simulink model "ML_UAV_3D_2"  (R2018a)
settings: Solver=ode4  StartTime=0.0  StopTime=130  FixedStep=Ts  MaxStep=2*T  MinStep=T  RelTol=1e-4
values from neighbouring files (symbols this model uses):
  Ac = 0.0331    [init_ML_UAV_3D_2.m]
  Am1_LPF = sysd.denominator{1}    [init_ML_UAV_3D_2.m]
  Am2_LPF = sysd.denominator{1}    [init_ML_UAV_3D_2.m]
  Am_coup_LPF = sysd.denominator{1}    [init_ML_UAV_3D_2.m]
  Amp_sf = 3    [init_ML_UAV_3D_2.m]
  Amp_sf_rp = 0.05*uav.m*g    [init_ML_UAV_3D_2.m]
  Bm1_LPF = sysd.numerator{1}    [init_ML_UAV_3D_2.m]
  Bm2_LPF = sysd.numerator{1}    [init_ML_UAV_3D_2.m]
  Bm_coup_LPF = sysd.numerator{1}    [init_ML_UAV_3D_2.m]
  C_S = [5;5;9]*10^-3    [init_ML_UAV_3D_2.m]
  Cd_u = 0.2    [init_ML_UAV_3D_2.m]
  dc_M_p = 6.7    [init_ML_UAV_3D_2.m]
  eps_V = 0.5    [init_ML_UAV_3D_2.m]
  g = 9.81    [init_ML_UAV_3D_2.m]
  gamma_d_p = (2*0.3/0.03*2*0.2*12/4)/10    (= 2.4)    [init_ML_UAV_3D_2.m]
  k3 = 24    [init_ML_UAV_3D_2.m]
  k4 = 0.8    [init_ML_UAV_3D_2.m]
  min_sf = 5    [init_ML_UAV_3D_2.m]
  min_sf_rp = 0.35*uav.m*g    [init_ML_UAV_3D_2.m]
  OMEGA_FILTER_OUTER = 40    [estimation.m]
  T_init = 10    [init_ML_UAV_3D_2.m]
  Tc = 1/500    (= 0.002)    [estimation.m]
  Tg = 1/ 20    (= 0.05)    [estimation.m]
  Tn = 1/500    (= 0.002)    [estimation.m]
  Ts = 1/500    (= 0.002)    [estimation.m]    (also in init_ML_UAV_3D_2.m)
  Tsc = 1/100    (= 0.01)    [estimation.m]
  Tz = 1/500    (= 0.002)    [estimation.m]
  X_GPS_offset = [0.01 0.005]    [estimation.m]
undefined symbols (not defined in the file or in its folder): Am_HPF, Am_LPF, Am_LPF2, an1, an1_v, an2, an3, Bm_HPF, Bm_LPF, Bm_LPF2, bn1, bn1_v, bn2, bn3, buoy, cable, controller, current, D_b, DiscIntNeverNeededParam, F, filters, J_u, K, kd_t, kp_t, L, Light, magnitude, MIL, Phi0, Psi0, R_b, T, Theta0, theta_q_ini, tolerences, torque_corr, uav, Vol_b, water, wave, X0_u
libraries: simulink x48, simulink_extras x10, UAV_Control x4, dspmtrx3 x2, aerolibwind2 x2
(part 1 of 6)
settings Model: Creator=Ahmad  LastModifiedBy=Ahmad
settings SolverCC: InitialStep=T  AlgebraicLoopSolver=LineSearch

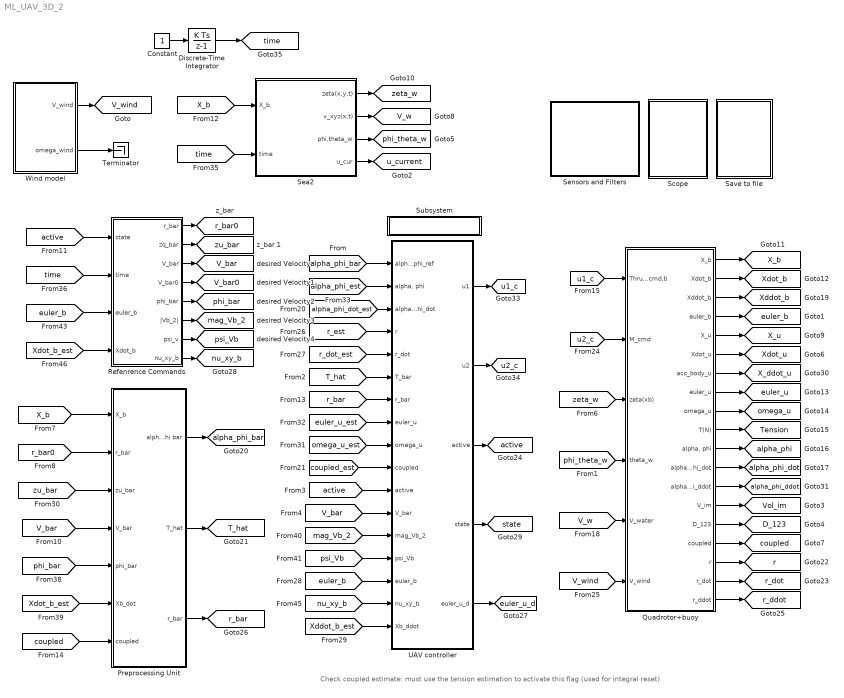
== system ML_UAV_3D_2 ==
  note: Check coupled estimate: must use the tension estimation to activate this flag (used for integral reset)
  Constant : Constant
  Discrete-Time Integrator : DiscreteIntegrator  SampleTime=Ts  ICPrevOutput=DiscIntNeverNeededParam  ICPrevScaledInput=DiscIntNeverNeededParam
  Preprocessing Unit : Subsystem
  Quadrotor+buoy : Subsystem
  Refenrence Commands : Subsystem
  Save to file : Subsystem
  Scope : Subsystem
  Sea2 : Subsystem
  Sensors and Filters : Subsystem
  Subsystem : Subsystem
      settings: OpenFcn=init_ML_UAV_3D_1
      mask Display:
      | text(.5,.5,'load parameters',...
      | 	'horizontalalignment','center');
  Terminator : Terminator
  UAV controller : Subsystem
  Wind model : Subsystem
  tag scope: D_123=global, T_hat=global, Tension=global, V_bar0=global, V_bar=global, V_w=global, V_wind=global, Vol_im=global, X_b=global, X_ddot_u=global, X_u=global, Xddot_b=global, Xdot_b=global, Xdot_u=global, active=global, alpha_phi=global, alpha_phi_bar=global, alpha_phi_ddot=global, alpha_phi_dot=global, coupled=global, euler_b=global, euler_u=global, euler_u_d=global, mag_Vb_2=global, nu_xy_b=global, omega_u=global, phi_bar=global, phi_theta_w=global, psi_Vb=global, r=global, r_bar0=global, r_bar=global, r_ddot=global, r_dot=global, state=global, time=global, u1_c=global, u2_c=global, u_current=global, zeta_w=global, zu_bar=global
  wires:
  [time] -> Sea2/2(time)
  [X_b] -> Sea2/1(X_b)
  Sea2/1(zeta(x,y,t)) -> [zeta_w]
  Sea2/2(v_xyz(x,t)) -> [V_w]
  Sea2/3(phi,theta_w) -> [phi_theta_w]
  [phi_theta_w] -> Quadrotor+buoy/4(theta_w)
  [V_w] -> Quadrotor+buoy/5(V_water)
  [zeta_w] -> Quadrotor+buoy/3(zeta(xb))
  Quadrotor+buoy/5(X_u) -> [X_u]
  Quadrotor+buoy/1(X_b) -> [X_b]
  Quadrotor+buoy/2(Xdot_b) -> [Xdot_b]
  Quadrotor+buoy/8(euler_u) -> [euler_u]
  Quadrotor+buoy/9(omega_u) -> [omega_u]
  Quadrotor+buoy/10(T(N)) -> [Tension]
  Quadrotor+buoy/11("alpha, phi") -> [alpha_phi]
  Quadrotor+buoy/12("alpha_dot, phi_dot") -> [alpha_phi_dot]
  [X_b] -> Preprocessing Unit/1(X_b)
  Preprocessing Unit/1("alpha, phi bar") -> [alpha_phi_bar]
  Preprocessing Unit/2(T_hat) -> [T_hat]
  Quadrotor+buoy/3(Xddot_b) -> [Xddot_b]
  Quadrotor+buoy/4(euler_b) -> [euler_b]
  Quadrotor+buoy/6(Xdot_u) -> [Xdot_u]
  Sea2/4(u_cur) -> [u_current]
  Quadrotor+buoy/14(V_im) -> [Vol_im]
  Quadrotor+buoy/15(D_123) -> [D_123]
  [alpha_phi_bar] -> UAV controller/1(alpha_phi_ref)
  [alpha_phi_est] -> UAV controller/2("alpha, phi")
  [alpha_phi_dot_est] -> UAV controller/3(alpha_phi_dot)
  [T_hat] -> UAV controller/6(T_bar)
  [Xddot_b_est] -> UAV controller/17(Xb_ddot)
  [euler_u_est] -> UAV controller/8(euler_u)
  [omega_u_est] -> UAV controller/9(omega_u)
  Quadrotor+buoy/16(coupled) -> [coupled]
  [active] -> Refenrence Commands/1(state)
  [r_bar] -> UAV controller/7(r_bar)
  Quadrotor+buoy/17(r) -> [r]
  Quadrotor+buoy/18(r_dot) -> [r_dot]
  [r_est] -> UAV controller/4(r)
  UAV controller/3(" active") -> [active]
  [active] -> UAV controller/11(active)
  [coupled_est] -> UAV controller/10(coupled)
  Quadrotor+buoy/19(r_ddot) -> [r_ddot]
  [r_dot_est] -> UAV controller/5(r_dot)
  Preprocessing Unit/3(" r_bar") -> [r_bar]
  UAV controller/4(state) -> [state]
  Quadrotor+buoy/7(acc_body_u) -> [X_ddot_u]
  Quadrotor+buoy/13("alpha_ddot, phi_ddot") -> [alpha_phi_ddot]
  Wind model/1(V_wind) -> [V_wind]
  Wind model/2(omega_wind) -> Terminator/1
  [V_wind] -> Quadrotor+buoy/6(V_wind)
  Refenrence Commands/1(r_bar) -> [r_bar0]
  [r_bar0] -> Preprocessing Unit/2(r_bar)
  Refenrence Commands/4(V_bar0) -> [V_bar0]
  Refenrence Commands/3(V_bar) -> [V_bar]
  [V_bar] -> Preprocessing Unit/4(V_bar)
  UAV controller/1(u1) -> [u1_c]
  UAV controller/2(u2) -> [u2_c]
  [u1_c] -> Quadrotor+buoy/1(Thrust_cmd,b)
  [u2_c] -> Quadrotor+buoy/2(M_cmd)
  Refenrence Commands/2(zq_bar) -> [zu_bar]
  [zu_bar] -> Preprocessing Unit/3(zu_bar)
  Constant/1 -> Discrete-Time Integrator/1
  Discrete-Time Integrator/1 -> [time]
  [time] -> Refenrence Commands/2(time)
  Refenrence Commands/5("phi_bar ") -> [phi_bar]
  [phi_bar] -> Preprocessing Unit/5(phi_bar)
  [Xdot_b_est] -> Preprocessing Unit/6(Xb_dot)
  Refenrence Commands/7(psi_v) -> [psi_Vb]
  Refenrence Commands/6(|Vb_2|) -> [mag_Vb_2]
  UAV controller/5(euler_u_d) -> [euler_u_d]
  [coupled] -> Preprocessing Unit/7(coupled)
  [psi_Vb] -> UAV controller/14(psi_Vb)
  [mag_Vb_2] -> UAV controller/13(mag_Vb_2)
  [euler_b] -> UAV controller/15(euler_b)
  [euler_b] -> Refenrence Commands/3(euler_b)
  Refenrence Commands/8(nu_xy_b) -> [nu_xy_b]
  [Xdot_b_est] -> Refenrence Commands/4(Xdot_b)
  [nu_xy_b] -> UAV controller/16(nu_xy_b)
  [V_bar] -> UAV controller/12(V_bar)

== system ML_UAV_3D_2/Preprocessing Unit ==
  X_b : Inport
  r_bar : Inport  Port=2
  zu_bar : Inport  Port=3
  V_bar : Inport  Port=4
  phi_bar : Inport  Port=5
  Xb_dot : Inport  Port=6
  coupled : Inport  Port=7
  Constant : Constant  Value=0
  Constant1 : Constant  Value=buoy.b_11
  Constant2 : Constant  Value=water.rho
  Constant3 : Constant  Value=water.nu
  Damping Coefficient Calculation : MATLAB Function  TreatAsAtomicUnit=on
  Dh @ no tension : Constant  Value=buoy.Delta_h
  Discrete Transfer Fcn1 : DiscreteTransferFcn  Numerator=filters.BmZ_LPF  Denominator=filters.AmZ_LPF  InitialStates=[1 1]*(1-sum(filters.AmZ_LPF))/(sum(filters.BmZ_LPF))*buoy.X0(3)
  Display : Display
  Display1 : Display
  Mux : Mux  Inputs=3
  Mux1 : Mux  Inputs=2
  Saturation : Saturate  UpperLimit=inf  LowerLimit=tolerences.epsilon_1
  Sum : Sum  Inputs=|+-
  Switch : Switch  Criteria=u2 > Threshold
  V_bar2 : InportShadow  Port=4
  alpha act vs des {,1..3} (4 alike) : Scope
  bottom plan : Constant  Value=buoy.h
  bottom plan1 : Constant  Value=buoy.l
  buoy elvation : Scope
  r_bar1 : InportShadow  Port=2
  "setpoint velocity controller " : MATLAB Function  TreatAsAtomicUnit=on
  smooth lower bound1 : Subsystem
  z_b : Selector  InputPortWidth=3  IndexOptions=Index vector (dialog)  Indices=3  OutputSizes=1
  "alpha, phi bar" : Outport
  T_hat : Outport  Port=2
  " r_bar" : Outport  Port=3
  wires:
  X_b/1 -> z_b/1
  zu_bar/1 -> alpha act vs des 1/1, "setpoint velocity controller "/6(zu_ref)
  Mux/1 -> buoy elvation/1
  Sum/1 -> Mux/3
  z_b/1 -> Discrete Transfer Fcn1/1, Mux/1, Sum/1
  Discrete Transfer Fcn1/1 -> "setpoint velocity controller "/5(zb), Mux/2, Sum/2  "better"
  r_bar1/1 -> " r_bar"/1
  Mux1/1 -> "alpha act vs des "/1, "alpha, phi bar"/1
  "setpoint velocity controller "/2(phi_bar_dec) -> Mux1/2
  [D11_0] -> "setpoint velocity controller "/7(D_b11)
  "setpoint velocity controller "/1(alpha_ref) -> Mux1/1
  phi_bar/1 -> alpha act vs des 3/1, "setpoint velocity controller "/2(phi_bar)
  V_bar/1 -> "setpoint velocity controller "/1(V_ref)
  Xb_dot/1 -> "setpoint velocity controller "/3(Vb)
  Saturation/1 -> smooth lower bound1/1(u)
  "setpoint velocity controller "/3(T_bar) -> Saturation/1
  smooth lower bound1/1(sat(u)) -> Switch/1
  Damping Coefficient Calculation/3(D11_0) -> [D11_0]
  Constant2/1 -> Damping Coefficient Calculation/5(rho)
  Constant1/1 -> Damping Coefficient Calculation/7(b_11)
  bottom plan/1 -> Damping Coefficient Calculation/3(h_b)
  bottom plan1/1 -> Damping Coefficient Calculation/4(l_b)
  Dh @ no tension/1 -> Damping Coefficient Calculation/2(delta_h)
  V_bar2/1 -> Damping Coefficient Calculation/1(V_bar)
  Constant3/1 -> Damping Coefficient Calculation/6(nu)
  r_bar/1 -> alpha act vs des 2/1, "setpoint velocity controller "/4(r_ref)
  Damping Coefficient Calculation/1(Re) -> Display/1
  Damping Coefficient Calculation/2(C_S_bar) -> Display1/1
  coupled/1 -> Switch/2
  Switch/1 -> T_hat/1
  Constant/1 -> Switch/3

== system ML_UAV_3D_2/Quadrotor+buoy ==
  Thrust_cmd,b : Inport
  M_cmd : Inport  Port=2
  zeta(xb) : Inport  Port=3
  theta_w : Inport  Port=4
  V_water : Inport  Port=5
  V_wind : Inport  Port=6
  6-DOF equations of motion Earth frame : Subsystem  mask(3DOF EoM, earth frame){pos_b_ini=buoy.X0, pos_u_ini=uav.X0, euler_b_ini=0, a_p_0=[uav.alpha_0; uav.phi_0], v_b_ini=buoy.V0, v_u_ini=uav.V0, euler_u_ini=uav.euler_0, omega_u_ini=0, m_u=1.7, J_u=uav.J, h_b=buoy.h, l_b=buoy.l, m_b=buoy.m, J_b=buoy.J, a_ii=[buoy.a_11 buoy.a_22  buoy.a_33], b_ii=[buoy.b_11 buoy.b_22 buoy.b_33 0 0 0], L=cable.L_0, g=g, rho_w=water.rho, coupled_ini=off}
      mask prompts: pos_b_ini "Buoy initial position (x y z):"; pos_u_ini "UAV initial position (x y z):"; euler_b_ini "Buoy initial body attitude:"; a_p_0 "Cable initial angle:"; v_b_ini "Buoy initial velocity (x y z):"; v_u_ini "UAV initial velocity (x y z):"; euler_u_ini "Quadrotor initial body attitude (quadrotor):"; omega_u_ini "Quadrotor initial body rotation rate:"; m_u "Quadrotor mass:"; J_u "Quadrotor moment of Inertia (3x3):"; h_b "Buoy height:"; l_b "Buoy lenght:"; m_b "Buoy mass:"; J_b "Buoy moment of Inertia (3x3):"; a_ii "Added mass (1x6):"; b_ii "Buoy damping coefficients (1x6):"; L "Cable length:"; g "gravity:"; rho_w "water density:"; coupled_ini "Initial coupling state (checked for coupled)"
      mask init:
      | nu_w = 1.787*10^-6;   % kinematic viscosity of water (m2/s)
      | g = 9.81;               % gravity constant (m/s2)
      | rho_w = 1000;   % water density (kg/m3)
      | rho_a = 1.225;             % air density (kg/m^3)
      | 
      | r_0 = norm(pos_u_ini - pos_b_ini);
      | 
      | R_S2C_0 = [cos(a_p_0(1))*cos(a_p_0(2))  -sin(a_p_0(1))*cos(a_p_0(2)) -sin(a_p_0(2))
      |            cos(a_p_0(1))*sin(a_p_0(2))  -sin(a_p_0(1))*sin(a_p_0(2))  cos(a_p_0(2))
      |            sin(a_p_0(1))                 cos(a_p_0(1))                0            ];
      |        
      | pos_u_0_coupled = pos_b_ini+L*[cos(a_p_0(1))*cos(a_p_0(2)); cos(a_p_0(1))*sin(a_p_0(2)); sin(a_p_0(1))];
      mask Display:
      | port_label('input',1,'u_1 (N)','texmode','on');
      | port_label('input',2,'\tau_{u,r} (N.m)','texmode','on');
      | port_label('input',3,'\zeta (m)','texmode','on');
      | port_label('input',4,'\phi_w,\theta_w (rad)','texmode','on');
      | port_label('input',5,'V_{water} (m/s)','texmode','on');
      | port_label('input',6,'V_{wind} (m/s)','texmode','on');
      | 
      | port_label('output',1,'X_b (m)','texmode','on');
      | port_label('output',2,'X_{b,dot} (m/s)','texmode','on');
      | port_label('output',3,'X_{b,ddot} (m/s)','texmode','on');
      | port_label('output',4,'euler_b(rad)','texmode','on');
      | port_label('output',5,'X_u (m)','texmode','on');
      | port_label('output',6,'X_{u,dot} (m/s)','texmode','on');
      | port_label('output',7,'X_{u,ddot} (m/s^2)','texmode','on');
      | port_label('output',8,'euler_u(rad)','texmode','on');
      | port_label('output',9,'\omega_u (rad/s)','texmode','on');
      | port_label('output',10,'\alpha, \phi (rad)','texmode','on');
      | port_label('output',11,'\alpha_{dot} \phi_{dot} (rad/s)','texmode','on');
      | port_label('output',12,'\alpha_{ddot} \phi_{ddot} (rad/s)','texmode','on');
      | port_label('output',13,'r (m)','texmode','on');
      | port_label('output',14,'r_{dot} (m/s)','texmode','on');
      | port_label('output',15,'r_{ddot} (m/s)','texmode','on');
      | port_label('output',16,'T (N)','texmode','on');
      | port_label('output',17,'V_{im} (m^3)','texmode','on');
      | port_label('output',18,'D_{123}','texmode','on');
      | port_label('output',19,'coupled','texmode','on');
  Gain : Gain
  Gain1 : Gain  Gain=[1 1 1]
  Mux : Mux  Inputs=2
  Mux1 : Mux  Inputs=2
  Saturation - Limit Height Controller1 : Saturate  UpperLimit=uav.K*uav.L*uav.torque_corr*[1 1 1]  LowerLimit=-uav.K*uav.L*uav.torque_corr*[1 1 1]
  Saturation - Limit Height Controller3 : Saturate  UpperLimit=uav.n_motors*uav.K  LowerLimit=0
  Signal Specification{,1..6,8} (8 alike) : SignalSpecification  Dimensions=[3,1]
  Signal Specification10 : SignalSpecification  Dimensions=[2,1]
  Signal Specification7 : SignalSpecification  Dimensions=[2,1]
  Signal Specification9 : SignalSpecification  Dimensions=[2,1]
  Torque : Scope
  "Xb " : Scope
  "Xq " : Scope
  motor dynamics (thrust) : DiscreteTransferFcn  Numerator=filters.Bm  Denominator=filters.Am  InitialStates=-filters.Am(2)/filters.Bm(2)*uav.m*g/cos(uav.euler_0(2))
  motor dynamics (torque) : DiscreteTransferFcn  Numerator=filters.Bm  Denominator=filters.Am
  thrust : Scope
  X_b : Outport
  Xdot_b : Outport  Port=2
  Xddot_b : Outport  Port=3
  euler_b : Outport  Port=4
  X_u : Outport  Port=5
  Xdot_u : Outport  Port=6
  acc_body_u : Outport  Port=7
  euler_u : Outport  Port=8
  omega_u : Outport  Port=9
  T(N) : Outport  Port=10
  "alpha, phi" : Outport  Port=11
  "alpha_dot, phi_dot" : Outport  Port=12
  "alpha_ddot, phi_ddot" : Outport  Port=13
  V_im : Outport  Port=14
  D_123 : Outport  Port=15
  coupled : Outport  Port=16
  r : Outport  Port=17
  r_dot : Outport  Port=18
  r_ddot : Outport  Port=19
  tag scope: tau_ur=global, u1=global
  wires:
  Saturation - Limit Height Controller3/1 -> Gain/1, Mux/2
  motor dynamics (torque)/1 -> Saturation - Limit Height Controller1/1
  M_cmd/1 -> Mux1/1, motor dynamics (torque)/1
  Thrust_cmd,b/1 -> Mux/1, motor dynamics (thrust)/1
  Saturation - Limit Height Controller1/1 -> Mux1/2, Gain1/1
  zeta(xb)/1 -> 6-DOF equations of motion Earth frame/3(zeta)
  theta_w/1 -> 6-DOF equations of motion Earth frame/4(phi_theta_w)
  V_water/1 -> 6-DOF equations of motion Earth frame/5(V_w)
  6-DOF equations of motion Earth frame/5(Xu) -> Signal Specification3/1  "X_u"
  6-DOF equations of motion Earth frame/1(Xb) -> Signal Specification/1  "X_b"
  6-DOF equations of motion Earth frame/2(Xb_dot) -> Signal Specification1/1  "Xdot_b"
  6-DOF equations of motion Earth frame/6(Xu_dot) -> Signal Specification4/1  "V_u"
  6-DOF equations of motion Earth frame/4(Attitude_buoy) -> euler_b/1  "euler_b"
  6-DOF equations of motion Earth frame/8(Attitude_quadrotor) -> Signal Specification6/1  "euler_u"
  6-DOF equations of motion Earth frame/9(omega_quadrotor) -> Signal Specification8/1  "omega_u"
  6-DOF equations of motion Earth frame/3(Xb_ddot) -> Signal Specification2/1
  motor dynamics (thrust)/1 -> Saturation - Limit Height Controller3/1
  6-DOF equations of motion Earth frame/11(alpha_phi_dot) -> Signal Specification9/1  "alpha_dot"
  6-DOF equations of motion Earth frame/16(Cable Tension) -> T(N)/1  "tension"
  6-DOF equations of motion Earth frame/10(alpha_phi) -> Signal Specification7/1  "alpha"
  Mux/1 -> thrust/1
  Mux1/1 -> Torque/1
  6-DOF equations of motion Earth frame/17(V_im) -> V_im/1
  Gain/1 -> 6-DOF equations of motion Earth frame/1(u1), [u1]
  Gain1/1 -> 6-DOF equations of motion Earth frame/2(tau_ur), [tau_ur]
  6-DOF equations of motion Earth frame/18("D_123 ") -> D_123/1
  6-DOF equations of motion Earth frame/19(coupled) -> coupled/1
  6-DOF equations of motion Earth frame/13("  r") -> r/1
  6-DOF equations of motion Earth frame/14("  rdot") -> r_dot/1
  6-DOF equations of motion Earth frame/15("  rddot") -> r_ddot/1
  6-DOF equations of motion Earth frame/7(Xu_ddot) -> Signal Specification5/1
  6-DOF equations of motion Earth frame/12(alpha_ddot) -> Signal Specification10/1
  V_wind/1 -> 6-DOF equations of motion Earth frame/6(V_wind)
  Signal Specification/1 -> "Xb "/1, X_b/1
  Signal Specification2/1 -> Xddot_b/1
  Signal Specification1/1 -> Xdot_b/1
  Signal Specification3/1 -> "Xq "/1, X_u/1
  Signal Specification5/1 -> acc_body_u/1
  Signal Specification4/1 -> Xdot_u/1
  Signal Specification6/1 -> euler_u/1
  Signal Specification8/1 -> omega_u/1
  Signal Specification7/1 -> "alpha, phi"/1
  Signal Specification10/1 -> "alpha_ddot, phi_ddot"/1
  Signal Specification9/1 -> "alpha_dot, phi_dot"/1

== system ML_UAV_3D_2/Refenrence Commands ==
  note: maybe you should start controlling the velocity imediatly and not wait for the uav to position itself in the expected final azimuth angleeventually the final azimuth angle could change and it is not efficient to follow it from the beginning.let the outer loop velocity controller work by itself.
  note: Smooth reference signals
  note: Initialization phase, reference r and zu
  note: Saturation protection
  note: V_r0_bar is the velocity of the buoy relative
      | to the water current (wave velocity is not included)
  state : Inport
  time : Inport  Port=2
  euler_b : Inport  Port=3
  Xdot_b : Inport  Port=4
  "  Vbar  " : Scope
  "  c" : Scope
  " r_ref " : Constant  Value=[uav.r_0 uav.r_bar]
  Bias : Bias  Bias=water.H+buoy.h/2
  Bias1 : Bias  Bias=-water.H-buoy.h/2
  Constant : Constant  Value=water.H
  Discrete Transfer Fcn (with initial outputs)1 : simulink_extras/Additional Discrete/Discrete Transfer Fcn (with initial outputs)  N=filters.Bm_rref_LPF  D=filters.Am_rref_LPF  U0=0  Y0=uav.r_0  TS=-1
      settings: SourceProductName=Simulink  SourceProductBaseCode=SL
  Discrete Transfer Fcn (with initial outputs)2 : simulink_extras/Additional Discrete/Discrete Transfer Fcn (with initial outputs)  N=filters.BmPsiV_LPF  D=filters.AmPsiV_LPF  U0=uav.phi_0  Y0=uav.phi_0  TS=-1
      settings: SourceProductName=Simulink  SourceProductBaseCode=SL
  Discrete Transfer Fcn (with initial outputs)3 : simulink_extras/Additional Discrete/Discrete Transfer Fcn (with initial outputs)  N=filters.BmV_LPF  D=filters.AmV_LPF  U0=0  Y0=0  TS=-1
      settings: SourceProductName=Simulink  SourceProductBaseCode=SL
  Discrete Transfer Fcn (with initial outputs)4 : simulink_extras/Additional Discrete/Discrete Transfer Fcn (with initial outputs)  N=filters.Bm_rref20_LPF  D=filters.Am_rref20_LPF  U0=0  Y0=uav.r_0  TS=-1
      settings: SourceProductName=Simulink  SourceProductBaseCode=SL
  From File : FromFile  Commented=on  FileName=Export\with waves\SVC\V_bar.mat  SampleTime=0
  From File1 : FromFile  Commented=on  FileName=Export\no waves\SVC\V_bar.mat  SampleTime=0
  From File2 : FromFile  Commented=on  FileName=Export\Monte Carlo\CM_21\SVCS\V_bar.mat  SampleTime=0
  Manual Switch1 : ManualSwitch  CurrentSetting=0
  Manual Switch2 : ManualSwitch  Commented=on
  Manual Switch4 : ManualSwitch
  Mux1 : Mux  Inputs=2
  Mux3 : Mux  Inputs=3
  "Rate Limiter for fly over test " : RateLimiter  RisingSlewLimit=2.5/10  FallingSlewLimit=-2.5/10  SampleTimeMode=inherited
  Saturation Dynamic : simulink/Discontinuities/Saturation Dynamic  OutMin=[]  OutMax=[]  OutDataTypeStr=Inherit: Same as second input  OutDataType=fixdt(1, 16)  OutScaling=2^-10  DoSatur=off
  Saturation Dynamic1 : simulink/Discontinuities/Saturation Dynamic  OutMin=[]  OutMax=[]  OutDataTypeStr=Inherit: Same as second input  OutDataType=fixdt(1, 16)  OutScaling=2^-10  DoSatur=off
  Scope1 : Scope
  Scope2 : Scope
  Selector1 : Selector  InputPortWidth=3  IndexOptions=Index vector (dialog)  Indices=[1,2]  OutputSizes=1
  Switch : Switch  Criteria=u2 > Threshold
  Switch4 : Switch  Criteria=u2 > Threshold
  V_ref : Constant  Value=[5 0+5 -5+10]
  cable length : Constant  Value=cable.L_0
  initialize r_bar : Step  Time=20  SampleTime=0
  minimum velocity error : Constant
  "psi_b " : Selector  InputPortWidth=3  IndexOptions=Index vector (dialog)  Indices=3  OutputSizes=1
  psi_v_ref : Constant  Value=[uav.phi_0*0 pi/2 pi]
  r error threshold [m] : Constant  Value=0.05
  r_ref for the coupled case (pulling) : Constant  Value=cable.L_0
  referense signals selector : MATLAB Function  TreatAsAtomicUnit=on
  setpoint velocity controller1 : MATLAB Function  TreatAsAtomicUnit=on
  smooth z_bar : simulink_extras/Additional Discrete/Discrete Transfer Fcn (with initial outputs)  N=filters.Bm_rref_LPF  D=filters.Am_rref_LPF  U0=uav.X0(3)-0.015  Y0=uav.X0(3)-0.015  TS=-1
      settings: SourceProductName=Simulink  SourceProductBaseCode=SL
  tr ref : Constant  Value=[0 1]
  tv_ref : Constant  Value=[T_init T_init+25 T_init+25+20]
  vector magnitude and angle1 : MATLAB Function  TreatAsAtomicUnit=on
  zu_ref : Constant  Value=[uav.X0(3)-0.015 uav.z_bar]
  r_bar : Outport
  zq_bar : Outport  Port=2
  V_bar : Outport  Port=3
  V_bar0 : Outport  Port=4
  "phi_bar " : Outport  Port=5
  |Vb_2| : Outport  Port=6
  psi_v : Outport  Port=7
  nu_xy_b : Outport  Port=8
  wires:
  referense signals selector/1(V_ref_out) -> setpoint velocity controller1/5(V0_bar), Mux3/3, V_bar0/1
  r_ref for the coupled case (pulling)/1 -> Switch/1, Saturation Dynamic1/1
  referense signals selector/3(r_ref_out) -> Switch/3  "r_ref when not 'pulling'"
  state/1 -> Switch/2
  Saturation Dynamic/1 -> Bias1/1, zq_bar/1
  Constant/1 -> Saturation Dynamic/3
  Bias/1 -> Saturation Dynamic/1
  Saturation Dynamic1/1 -> r_bar/1
  Bias1/1 -> Saturation Dynamic1/3
  smooth z_bar/1 -> Saturation Dynamic/2
  Switch4/1 -> Bias/1, Saturation Dynamic1/2  "r_bar"
  referense signals selector/4(zu_ref_out) -> smooth z_bar/1
  Switch/1 -> Discrete Transfer Fcn (with initial outputs)1/1, Discrete Transfer Fcn (with initial outputs)4/1
  minimum velocity error/1 -> setpoint velocity controller1/1(eps)
  [r_est] -> setpoint velocity controller1/2(r)
  r error threshold [m]/1 -> setpoint velocity controller1/3(er_thr)
  cable length/1 -> setpoint velocity controller1/4(Lc0)
  Xdot_b/1 -> Selector1/1
  setpoint velocity controller1/3(c) -> "  c"/1
  Discrete Transfer Fcn (with initial outputs)3/1 -> Manual Switch1/2, Mux3/1
  Mux3/1 -> "  Vbar  "/1
  initialize r_bar/1 -> Switch4/2
  Discrete Transfer Fcn (with initial outputs)4/1 -> Switch4/1
  Discrete Transfer Fcn (with initial outputs)1/1 -> Switch4/3
  Manual Switch1/1 -> V_bar/1
  From File/1 -> Manual Switch2/2
  From File1/1 -> Manual Switch2/1
  Manual Switch4/1 -> Discrete Transfer Fcn (with initial outputs)3/1, Mux3/2
  setpoint velocity controller1/1(V_bar_out) -> "Rate Limiter for fly over test "/1, Manual Switch4/1
  "Rate Limiter for fly over test "/1 -> Manual Switch4/2
  From File2/1 -> Manual Switch1/1
  time/1 -> referense signals selector/7(t)
  " r_ref "/1 -> referense signals selector/4(r_ref)
  tr ref/1 -> referense signals selector/6(tr_ref)
  zu_ref/1 -> referense signals selector/5(zu_ref)
  tv_ref/1 -> referense signals selector/3(tv_ref)
  V_ref/1 -> referense signals selector/1(V_ref)
  psi_v_ref/1 -> referense signals selector/2(phi_ref)
  referense signals selector/2(phi_ref_out) -> setpoint velocity controller1/6(phi0_bar)
  Selector1/1 -> Scope1/1, vector magnitude and angle1/1(U2)
  vector magnitude and angle1/2(direction2) -> Scope2/1, psi_v/1
  setpoint velocity controller1/2(phi_bar_out) -> Discrete Transfer Fcn (with initial outputs)2/1
  Discrete Transfer Fcn (with initial outputs)2/1 -> "phi_bar "/1
  euler_b/1 -> "psi_b "/1
  "psi_b "/1 -> vector magnitude and angle1/2(psi_b)
  vector magnitude and angle1/3(nu_xb) -> setpoint velocity controller1/7(V), Mux1/1
  vector magnitude and angle1/4(nu_yb) -> Mux1/2
  Mux1/1 -> nu_xy_b/1
  vector magnitude and angle1/1(mag_u2) -> |Vb_2|/1

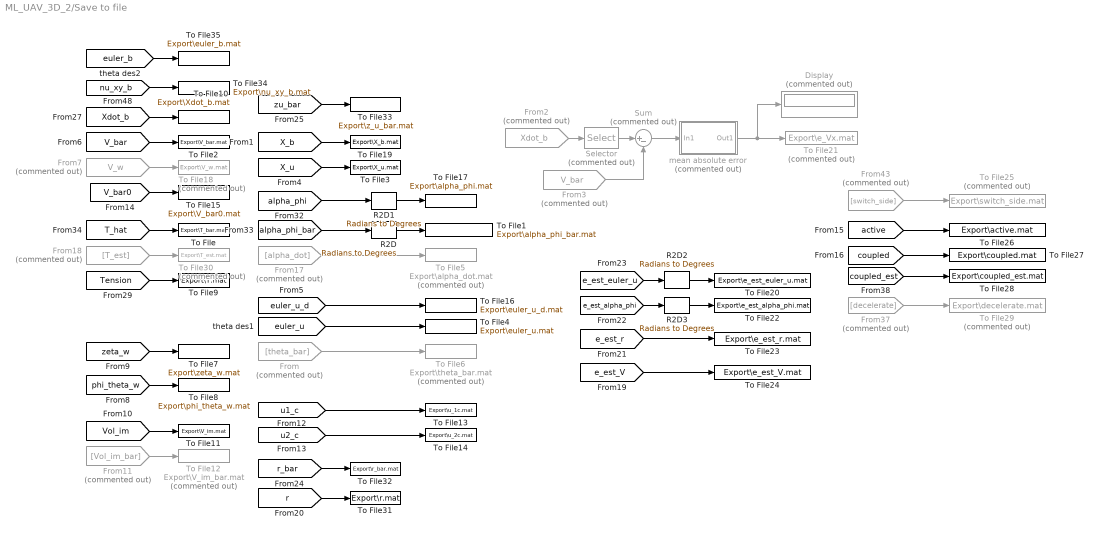
== system ML_UAV_3D_2/Save to file ==
  Display : Display  Commented=on
  From : From  Commented=on  GotoTag=theta_bar  TagVisibility=global
  From11 : From  Commented=on  GotoTag=Vol_im_bar
  From17 : From  Commented=on  GotoTag=alpha_dot  TagVisibility=global
  From18 : From  Commented=on  GotoTag=T_est
  From2 : From  Commented=on  GotoTag=Xdot_b  TagVisibility=global
  From3 : From  Commented=on  GotoTag=V_bar  TagVisibility=global
  From37 : From  Commented=on  GotoTag=decelerate  TagVisibility=global
  From43 : From  Commented=on  GotoTag=switch_side
  From7 : From  Commented=on  GotoTag=V_w  TagVisibility=global
  R2D{,1..3} (4 alike) : simulink_extras/Transformations/Radians to Degrees
  Selector : Selector  Commented=on  InputPortWidth=2  IndexOptions=Index vector (dialog)  Indices=1  OutputSizes=1
  Sum : Sum  Commented=on  Inputs=|+-
  To File : ToFile  Filename=Export\T_bar.mat  MatrixName=T_bar  SaveFormat=Timeseries  SampleTime=floor(Ts/4)
  To File1 : ToFile  Filename=Export\alpha_phi_bar.mat  MatrixName=alpha_phi_bar  SaveFormat=Timeseries  SampleTime=floor(Ts/4)
  To File10 : ToFile  Filename=Export\Xdot_b.mat  MatrixName=Xdot_b  SaveFormat=Timeseries  SampleTime=floor(Ts/4)
  To File11 : ToFile  Filename=Export\V_im.mat  MatrixName=V_im  SaveFormat=Timeseries  SampleTime=floor(Ts/4)
  To File12 : ToFile  Commented=on  Filename=Export\V_im_bar.mat  MatrixName=V_im_bar  SaveFormat=Timeseries  SampleTime=floor(Ts/4)
  To File13 : ToFile  Filename=Export\u_1c.mat  MatrixName=u_1c  SaveFormat=Timeseries  SampleTime=floor(Ts/4)
  To File14 : ToFile  Filename=Export\u_2c.mat  MatrixName=u_2c  SaveFormat=Timeseries  SampleTime=floor(Ts/4)
  To File15 : ToFile  Filename=Export\V_bar0.mat  MatrixName=V_bar0  SaveFormat=Timeseries  SampleTime=floor(Ts/4)
  To File16 : ToFile  Filename=Export\euler_u_d.mat  MatrixName=euler_u_d  SaveFormat=Timeseries  SampleTime=floor(Ts/4)
  To File17 : ToFile  Filename=Export\alpha_phi.mat  MatrixName=alpha_phi  SaveFormat=Timeseries  SampleTime=floor(Ts/4)
  To File18 : ToFile  Commented=on  Filename=Export\V_w.mat  MatrixName=V_w  SaveFormat=Timeseries  SampleTime=floor(T/4)
  To File19 : ToFile  Filename=Export\X_b.mat  MatrixName=X_b  SaveFormat=Timeseries  SampleTime=floor(Ts/4)
  To File2 : ToFile  Filename=Export\V_bar.mat  MatrixName=V_bar  SaveFormat=Timeseries  SampleTime=floor(Ts/4)
  To File20 : ToFile  Filename=Export\e_est_euler_u.mat  MatrixName=e_est_euler_u  SaveFormat=Timeseries  SampleTime=floor(Ts/4)
  To File21 : ToFile  Commented=on  Filename=Export\e_Vx.mat  MatrixName=Vx  SaveFormat=Timeseries  SampleTime=floor(T/4)
  To File22 : ToFile  Filename=Export\e_est_alpha_phi.mat  MatrixName=e_est_alpha_phi  SaveFormat=Timeseries  SampleTime=floor(Ts/4)
  To File23 : ToFile  Filename=Export\e_est_r.mat  MatrixName=e_est_r  SaveFormat=Timeseries  SampleTime=floor(Ts/4)
  To File24 : ToFile  Filename=Export\e_est_V.mat  MatrixName=e_est_V  SaveFormat=Timeseries  SampleTime=floor(Ts/4)
  To File25 : ToFile  Commented=on  Filename=Export\switch_side.mat  MatrixName=switch_side  SaveFormat=Timeseries  SampleTime=floor(Ts/4)
  To File26 : ToFile  Filename=Export\active.mat  MatrixName=active  SaveFormat=Timeseries  SampleTime=floor(Ts/4)
  To File27 : ToFile  Filename=Export\coupled.mat  MatrixName=coupled  SaveFormat=Timeseries  SampleTime=floor(Ts/4)
  To File28 : ToFile  Filename=Export\coupled_est.mat  MatrixName=coupled_est  SaveFormat=Timeseries  SampleTime=floor(Ts/4)
  To File29 : ToFile  Commented=on  Filename=Export\decelerate.mat  MatrixName=decelerate  SaveFormat=Timeseries  SampleTime=floor(T/4)
  To File3 : ToFile  Filename=Export\X_u.mat  MatrixName=X_u  SaveFormat=Timeseries  SampleTime=floor(Ts/4)
  To File30 : ToFile  Commented=on  Filename=Export\T_est.mat  MatrixName=T_est  SaveFormat=Timeseries  SampleTime=floor(Ts/4)
  To File31 : ToFile  Filename=Export\r.mat  MatrixName=r  SaveFormat=Timeseries  SampleTime=floor(Ts/4)
  To File32 : ToFile  Filename=Export\r_bar.mat  MatrixName=r_bar  SaveFormat=Timeseries  SampleTime=floor(Ts/4)
  To File33 : ToFile  Filename=Export\z_u_bar.mat  MatrixName=z_u_bar  SaveFormat=Timeseries  SampleTime=floor(Ts/4)
  To File34 : ToFile  Filename=Export\nu_xy_b.mat  MatrixName=nu_xy_b  SaveFormat=Timeseries  SampleTime=floor(Ts/4)
  To File35 : ToFile  Filename=Export\euler_b.mat  MatrixName=euler_b  SaveFormat=Timeseries  SampleTime=floor(Ts/4)
  To File4 : ToFile  Filename=Export\euler_u.mat  MatrixName=euler_u  SaveFormat=Timeseries  SampleTime=floor(Ts/4)
  To File5 : ToFile  Commented=on  Filename=Export\alpha_dot.mat  MatrixName=alpha_dot  SaveFormat=Timeseries  SampleTime=floor(T/4)
  To File6 : ToFile  Commented=on  Filename=Export\theta_bar.mat  MatrixName=theta_bar  SaveFormat=Timeseries  SampleTime=floor(T/4)
  To File7 : ToFile  Filename=Export\zeta_w.mat  MatrixName=zeta_w  SaveFormat=Timeseries  SampleTime=floor(Ts/4)
  To File8 : ToFile  Filename=Export\phi_theta_w.mat  MatrixName=phi_theta_w  SaveFormat=Timeseries  SampleTime=floor(Ts/4)
  To File9 : ToFile  Filename=Export\T.mat  MatrixName=T  SaveFormat=Timeseries  SampleTime=floor(Ts/4)
  mean absolute error : Subsystem  Commented=on
  wires:
  R2D/1 -> To File1/1
  [X_u] -> To File3/1
  [alpha_phi_bar] -> R2D/1
  [V_bar] -> To File2/1
  [euler_u_d] -> To File16/1
  [alpha_phi] -> R2D1/1
  R2D1/1 -> To File17/1
  From7/1 -> To File18/1
  [X_b] -> To File19/1
  Sum/1 -> mean absolute error/1(In1)
  mean absolute error/1(Out1) -> Display/1, To File21/1
  [T_hat] -> To File/1
  [euler_u] -> To File4/1
  From17/1 -> To File5/1
  From/1 -> To File6/1
  [zeta_w] -> To File7/1
  [phi_theta_w] -> To File8/1
  [Tension] -> To File9/1
  [Xdot_b] -> To File10/1
  From2/1 -> Selector/1
  From3/1 -> Sum/2
  Selector/1 -> Sum/1
  [Vol_im] -> To File11/1
  From11/1 -> To File12/1
  [u1_c] -> To File13/1
  [u2_c] -> To File14/1
  [V_bar0] -> To File15/1
  [e_est_euler_u] -> R2D2/1
  R2D2/1 -> To File20/1
  [e_est_alpha_phi] -> R2D3/1
  R2D3/1 -> To File22/1
  [e_est_r] -> To File23/1
  [e_est_V] -> To File24/1
  From43/1 -> To File25/1
  [active] -> To File26/1
  [coupled] -> To File27/1
  [coupled_est] -> To File28/1
  From37/1 -> To File29/1
  From18/1 -> To File30/1
  [r] -> To File31/1
  [r_bar] -> To File32/1
  [zu_bar] -> To File33/1
  [nu_xy_b] -> To File34/1
  [euler_b] -> To File35/1

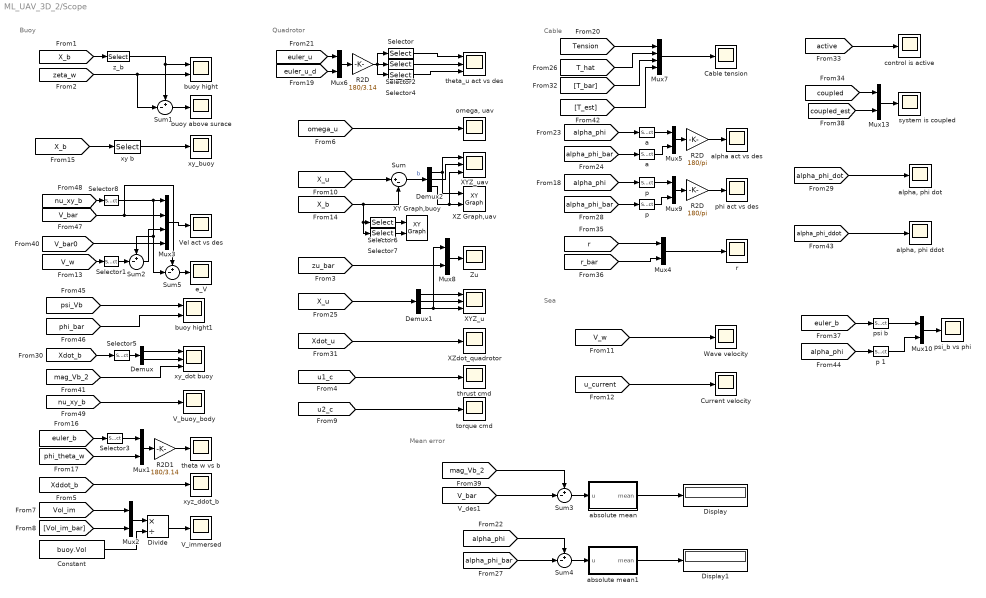
== system ML_UAV_3D_2/Scope ==
  note: Mean error
  note: Sea
  note: Cable
  note: Quadrotor
  note: Buoy
  " a" : Selector  InputPortWidth=2  IndexOptions=Index vector (dialog)  Indices=1  OutputSizes=1
  " p" : Selector  InputPortWidth=2  IndexOptions=Index vector (dialog)  Indices=2  OutputSizes=1
  " r" : Scope
  Cable tension : Scope
  Constant : Constant  Value=buoy.Vol
  Current velocity : Scope
  Demux : Demux  Outputs=2
  Demux1 : Demux  Outputs=3
  Demux2 : Demux  Outputs=3
  Display : Display
  Display1 : Display
  Divide : Product  Inputs=*/
  Mux{1..2,4..6,8..10,13} (9 alike) : Mux  Inputs=2
  Mux3 : Mux
  Mux7 : Mux
  R2D : Gain  Gain=180/3.14
  "R2D " : Gain  Gain=180/pi
  "R2D  " : Gain  Gain=180/pi
  R2D1 : Gain  Gain=180/3.14
  Selector : Selector  InputPortWidth=6  IndexOptions=Index vector (dialog)  Indices=[1 4]  OutputSizes=1
  Selector1 : Selector  InputPortWidth=3  IndexOptions=Index vector (dialog)  Indices=1  OutputSizes=1
  Selector2 : Selector  InputPortWidth=6  IndexOptions=Index vector (dialog)  Indices=[2 5]  OutputSizes=1
  Selector3 : Selector  InputPortWidth=3  IndexOptions=Index vector (dialog)  Indices=[1 2]  OutputSizes=1
  Selector4 : Selector  InputPortWidth=6  IndexOptions=Index vector (dialog)  Indices=[3 6]  OutputSizes=1
  Selector5 : Selector  InputPortWidth=3  IndexOptions=Index vector (dialog)  Indices=[1 2]  OutputSizes=1
  Selector6 : Selector  InputPortWidth=3  IndexOptions=Index vector (dialog)  Indices=1  OutputSizes=1
  Selector7 : Selector  InputPortWidth=3  IndexOptions=Index vector (dialog)  Indices=2  OutputSizes=1
  Selector8 : Selector  InputPortWidth=2  IndexOptions=Index vector (dialog)  Indices=1  OutputSizes=1
  Sum : Sum  Inputs=|+-
  Sum{1..5} (5 alike) : Sum  Inputs=+-|
  V_buoy_body : Scope
  V_immersed : Scope
  Vel act vs des : Scope
  Wave velocity : Scope
  XY Graph,buoy : simulink/Sinks/XY Graph  xmin=-20  xmax=500  ymin=-20  ymax=500  st=1/10
  XYZ_u : Scope  NumInputPorts=3
  XYZ_uav : Scope  NumInputPorts=3
  XZ Graph,uav : simulink/Sinks/XY Graph  xmin=-17  xmax=17  ymin=0  ymax=17  st=1/10
  XZdot_quadrotor : Scope
  Zu : Scope
  "a " : Selector  InputPortWidth=2  IndexOptions=Index vector (dialog)  Indices=1  OutputSizes=1
  absolute mean : Subsystem
  absolute mean1 : Subsystem
  "alpha act vs des " : Scope
  "alpha, phi ddot" : Scope
  "alpha, phi dot" : Scope
  buoy above surace : Scope
  buoy hight : Scope  NumInputPorts=2
  buoy hight1 : Scope  NumInputPorts=2
  control is active : Scope
  e_V : Scope
  "omega, uav" : Scope
  "p " : Selector  InputPortWidth=2  IndexOptions=Index vector (dialog)  Indices=2  OutputSizes=1
  p 1 : Selector  InputPortWidth=2  IndexOptions=Index vector (dialog)  Indices=2  OutputSizes=1
  "phi act vs des " : Scope
  "psi b " : Selector  InputPortWidth=3  IndexOptions=Index vector (dialog)  Indices=3  OutputSizes=1
  psi_b vs phi : Scope
  system is coupled : Scope
  theta w vs b : Scope
  theta_u act vs des : Scope  NumInputPorts=3
  thrust cmd : Scope
  torque cmd : Scope
  xy b : Selector  InputPortWidth=3  IndexOptions=Index vector (dialog)  Indices=[1 2]  OutputSizes=1
  xy_buoy : Scope
  xy_dot buoy : Scope  NumInputPorts=3
  xyz_ddot_b : Scope
  z_b : Selector  InputPortWidth=3  IndexOptions=Index vector (dialog)  Indices=3  OutputSizes=1
  wires:
  z_b/1 -> Sum1/1, buoy hight/1
  [zeta_w] -> Sum1/2, buoy hight/2
  [omega_u] -> "omega, uav"/1
  [X_b] -> Selector7/1, Selector6/1, Sum/2
  Sum/1 -> Demux2/1  "b"
  [X_b] -> z_b/1
  Sum1/1 -> buoy above surace/1
  Mux1/1 -> R2D1/1
  Mux6/1 -> R2D/1
  Mux7/1 -> Cable tension/1
  Demux2/3 -> XYZ_uav/3, XZ Graph,uav/2
  Demux2/1 -> XYZ_uav/1, XZ Graph,uav/1
  [V_bar] -> Sum5/1, Mux3/2
  [euler_u_d] -> Mux6/2
  [euler_u] -> Mux6/1
  Mux3/1 -> Vel act vs des/1
  [alpha_phi] -> "a "/1
  [alpha_phi_bar] -> " a"/1
  Mux5/1 -> "R2D "/1
  [X_u] -> Sum/1
  [X_u] -> Demux1/1
  [nu_xy_b] -> Selector8/1
  "R2D "/1 -> "alpha act vs des "/1
  [Tension] -> Mux7/1
  [T_hat] -> Mux7/2
  [X_b] -> xy b/1
  xy b/1 -> xy_buoy/1
  [Xddot_b] -> xyz_ddot_b/1
  [Vol_im] -> Mux2/1
  [Vol_im_bar] -> Mux2/2
  Divide/1 -> V_immersed/1
  R2D1/1 -> theta w vs b/1
  Mux2/1 -> Divide/1
  Constant/1 -> Divide/2
  [u1_c] -> thrust cmd/1
  [u2_c] -> torque cmd/1
  [V_w] -> Wave velocity/1
  [u_current] -> Current velocity/1
  Demux1/2 -> XYZ_u/2
  Demux1/1 -> XYZ_u/1
  [V_w] -> Selector1/1
  Sum2/1 -> Mux3/3
  Selector1/1 -> Sum2/2
  [V_bar] -> Sum3/2
  [mag_Vb_2] -> Sum3/1
  Sum3/1 -> absolute mean/1(u)
  absolute mean/1(mean) -> Display/1
  [alpha_phi] -> Sum4/1
  [alpha_phi_bar] -> Sum4/2
  Sum4/1 -> absolute mean1/1(u)
  absolute mean1/1(mean) -> Display1/1
  [T_bar] -> Mux7/3
  [Xdot_u] -> XZdot_quadrotor/1
  [active] -> control is active/1
  [coupled] -> Mux13/1
  [r] -> Mux4/1
  Mux4/1 -> " r"/1
  [r_bar] -> Mux4/2
  [coupled_est] -> Mux13/2
  Mux13/1 -> system is coupled/1
  Sum5/1 -> e_V/1
  [zu_bar] -> Mux8/2
  Mux8/1 -> Zu/1
  [T_est] -> Mux7/4
  [V_bar0] -> Mux3/4
  [psi_Vb] -> buoy hight1/1
  [phi_bar] -> buoy hight1/2
  [phi_theta_w] -> Mux1/2
  [euler_b] -> Selector3/1
  Selector3/1 -> Mux1/1
  Demux1/3 -> Mux8/1, XYZ_u/3
  [alpha_phi] -> "p "/1
  Mux9/1 -> "R2D  "/1
  [alpha_phi_bar] -> " p"/1
  "R2D  "/1 -> "phi act vs des "/1
  "p "/1 -> Mux9/1
  " p"/1 -> Mux9/2
  "a "/1 -> Mux5/1
  " a"/1 -> Mux5/2
  Selector/1 -> theta_u act vs des/1
  Selector2/1 -> theta_u act vs des/2
  Selector4/1 -> theta_u act vs des/3
  R2D/1 -> Selector/1, Selector4/1, Selector2/1
  Demux2/2 -> XYZ_uav/2
  [alpha_phi_dot] -> "alpha, phi dot"/1
  [alpha_phi_ddot] -> "alpha, phi ddot"/1
  [Xdot_b] -> Selector5/1
  Demux/2 -> xy_dot buoy/2
  Demux/1 -> xy_dot buoy/1
  Selector5/1 -> Demux/1
  [alpha_phi] -> p 1/1
  [euler_b] -> "psi b "/1
  "psi b "/1 -> Mux10/1
  p 1/1 -> Mux10/2
  Mux10/1 -> psi_b vs phi/1
  Selector6/1 -> XY Graph,buoy/1
  Selector7/1 -> XY Graph,buoy/2
  Selector8/1 -> Sum5/2, Sum2/1, Mux3/1
  [mag_Vb_2] -> xy_dot buoy/3
  [nu_xy_b] -> V_buoy_body/1

== system ML_UAV_3D_2/Sea2 ==
  X_b : Inport
  time : Inport  Port=2
  Constant : Constant  Value=current.total
  Constant20 : Constant  Value=wave.A
  Constant21 : Constant  Value=wave.psi
  Constant22 : Constant  Value=wave.omega
  Constant23 : Constant  Value=wave.k
  Constant24 : Constant  Value=wave.epsilon
  Constant3 : Constant  Value=current.beta
  Constant4 : Constant  Value=wave.psi
  Constant5 : Constant  Value=wave.StocksDrift
  Constant6 : Constant  Value=water.H
  Demux3 : Demux  Outputs=3
  Ground : Ground
  Mean water level1 : Bias  Bias=water.H
  Mux : Mux  Inputs=3
  Mux1 : Mux  Inputs=2
  Mux2 : Mux  Inputs=3
  Sum : Sum  Inputs=|++
  Sum10 : Sum  Inputs=|++
  Sum11 : Sum  Inputs=|+-
  Sum9 : Sum  Inputs=|++
  Water current : MATLAB Function  TreatAsAtomicUnit=on
  Waves (elevation and speed) : MATLAB Function  TreatAsAtomicUnit=on
  psi : Selector  InputPortWidth=3  IndexOptions=Index vector (dialog)  Indices=3  OutputSizes=1
  zeta(x,y,t) : Outport
  v_xyz(x,t) : Outport  Port=2
  phi,theta_w : Outport  Port=3
  u_cur : Outport  Port=4
  wires:
  X_b/1 -> Demux3/1
  Constant20/1 -> Waves (elevation and speed)/5(A)
  Demux3/2 -> Waves (elevation and speed)/2(y)
  Constant22/1 -> Waves (elevation and speed)/7(omega)
  Demux3/1 -> Waves (elevation and speed)/1(x)
  Constant24/1 -> Waves (elevation and speed)/9(epsilon)
  Constant21/1 -> Waves (elevation and speed)/6(psi)
  time/1 -> Waves (elevation and speed)/4(t)
  Constant23/1 -> Waves (elevation and speed)/8(k)
  Constant/1 -> Water current/1(Uc)
  Constant3/1 -> Water current/3(beta)
  Constant4/1 -> Water current/5(psi_w)
  Constant5/1 -> Water current/2(Us)
  [euler_b] -> psi/1
  psi/1 -> Water current/4(psi_b)
  Waves (elevation and speed)/1(zeta_xy) -> Mean water level1/1
  Mux/1 -> v_xyz(x,t)/1
  Sum/1 -> Mux/1
  Sum10/1 -> Mux/3
  Sum9/1 -> Mux/2
  Water current/1(uc) -> Sum/1, Mux2/1
  Water current/2(vc) -> Mux2/2, Sum9/1
  Waves (elevation and speed)/2(uw) -> Sum/2
  Waves (elevation and speed)/3(vw) -> Sum9/2
  Waves (elevation and speed)/4(ww) -> Sum10/2
  Waves (elevation and speed)/5(phi_water) -> Mux1/1
  Waves (elevation and speed)/6(theta_water) -> Mux1/2
  Mux1/1 -> phi,theta_w/1
  Ground/1 -> Mux2/3, Sum10/1
  Constant6/1 -> Sum11/2
  Demux3/3 -> Sum11/1
  Sum11/1 -> Waves (elevation and speed)/3(z)
  Mean water level1/1 -> zeta(x,y,t)/1
  Mux2/1 -> u_cur/1

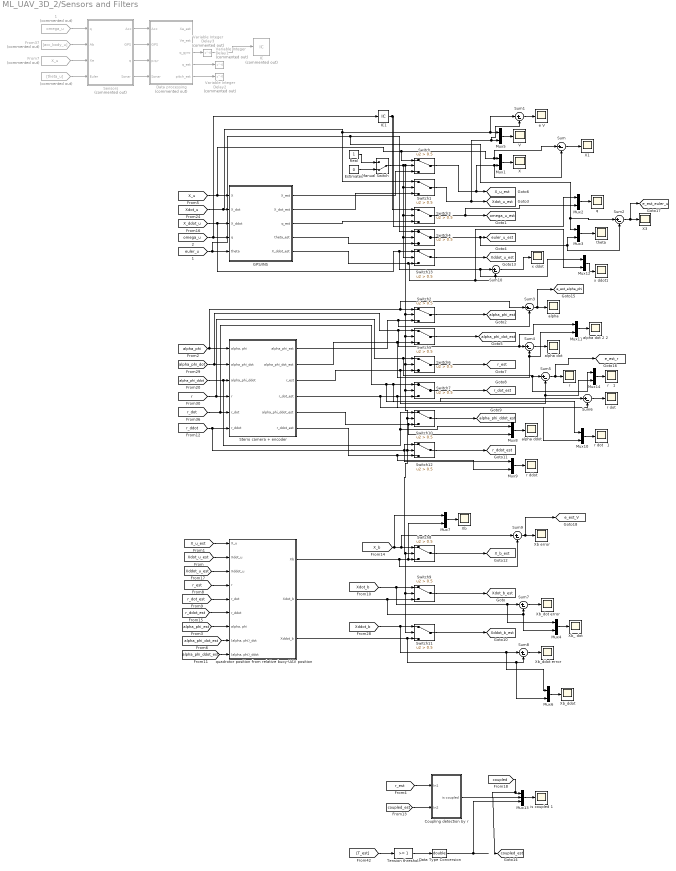
== system ML_UAV_3D_2/Sensors and Filters ==
  "    " : From  Commented=on  GotoTag=theta_u  TagVisibility=global
  "   1" : From  Commented=on  GotoTag=omega_u  TagVisibility=global
  Coupling detection by r : Subsystem
  Data Type Conversion : DataTypeConversion  OutDataTypeStr=double
  Data processing : Subsystem  Commented=on
  Estimates : Constant  Value=0
  From37 : From  Commented=on  GotoTag=acc_body_u  TagVisibility=global
  From7 : From  Commented=on  GotoTag=X_u  TagVisibility=global
  GPS/INS : Subsystem
  IC : InitialCondition  Commented=on  Value=0
  IC1 : InitialCondition  Value=0
  Manual Switch : ManualSwitch  CurrentSetting=0
  Mux{1..12,14} (13 alike) : Mux  Inputs=2
  Mux13 : Mux  Inputs=3
  Real : Constant
  Sensors : Subsystem  Commented=on
  Sterio camera + encoder : Subsystem
  Sum{,1..10} (11 alike) : Sum  Inputs=|+-
  Switch{,1..13} (14 alike) : Switch  Criteria=u2 > Threshold  Threshold=0.5
  Tension threshold : simulink/Logic and Bit Operations/Compare To Constant  relop=>=  const=1  OutDataTypeStr=boolean
  V : Scope
  Variable Integer Delay1 : Delay  Commented=on  DelayLength=0
  Variable Integer Delay2 : Delay  Commented=on  DelayLength=0
  Variable Integer Delay3 : Delay  Commented=on  DelayLength=0
  X : Scope
  X1 : Scope
  X3 : Scope
  "Xb " : Scope
  Xb error : Scope
  "Xb_ dot " : Scope
  "Xb_ddot " : Scope
  "Xb_ddot error  " : Scope
  Xb_dot error : Scope
  "alpha  " : Scope
  "alpha ddot " : Scope
  "alpha dot " : Scope
  alpha dot 2 2 : Scope
  e V : Scope
  is coupled 1 : Scope
  q : Scope
  quadrotor position from relative buoy-UAV position : Subsystem
  "r   " : Scope
  r   1 : Scope
  "r ddot   " : Scope
  "r dot  " : Scope
  r dot   1 : Scope
  theta : Scope
  x ddot : Scope
  x ddot1 : Scope
  tag scope: X_b_est=global, X_u_est=global, Xddot_b_est=global, Xddot_u_est=global, Xdot_b_est=global, Xdot_u_est=global, alpha_phi_ddot_est=global, alpha_phi_dot_est=global, alpha_phi_est=global, coupled_est=global, e_est_V=global, e_est_alpha_phi=global, e_est_euler_u=global, e_est_r=global, euler_u_est=global, omega_u_est=global, r_ddot_est=global, r_dot_est=global, r_est=global
  wires:
  Data processing/4("q_est ") -> Variable Integer Delay1/1
  "    "/1 -> Sensors/4(Euler)
  Sensors/3(" q") -> Data processing/3(p,q,r)
  "   1"/1 -> Sensors/1("q ")
  From7/1 -> Sensors/3(Xe)
  Sensors/1(Acc) -> Data processing/1(Acc)
  Sensors/2(GPS) -> Data processing/2("GPS ")
  From37/1 -> Sensors/2(Ab)
  Data processing/3(q_gyro) -> Variable Integer Delay3/1
  Data processing/5(pitch_est) -> Variable Integer Delay2/1
  Sensors/4(Sonar) -> Data processing/4(Sonar)
  Estimates/1 -> Manual Switch/2
  Real/1 -> Manual Switch/1
  Switch/1 -> Sum/2, Mux1/2, [X_u_est]
  Switch1/1 -> Sum1/2, Mux5/2, [Xdot_u_est]
  Switch3/1 -> Mux2/2, [omega_u_est]
  Switch4/1 -> Mux3/2, Sum2/2, [euler_u_est]
  GPS/INS/1(X_est) -> Switch/3
  GPS/INS/2(X_dot_est) -> Switch1/3
  Variable Integer Delay3/1 -> IC/1
  [X_u] -> Sum/1, Mux1/1, Switch/1, GPS/INS/1(X)
  [omega_u] -> IC1/1, GPS/INS/4(q)
  [Xdot_u] -> Sum1/1, Mux5/1, Switch1/1, GPS/INS/2(X_dot)
  GPS/INS/4(theta_est) -> Switch4/3
  GPS/INS/3(q_est) -> Switch3/3
  IC1/1 -> Mux2/1, Switch3/1
  [euler_u] -> Sum2/1, Mux3/1, Switch4/1, GPS/INS/5(theta)
  Mux5/1 -> V/1
  Mux1/1 -> X/1
  Mux2/1 -> q/1
  Mux3/1 -> theta/1
  Sum/1 -> X1/1
  Sum1/1 -> e V/1
  Sum2/1 -> [e_est_euler_u], X3/1
  [alpha_phi_dot] -> Mux11/1, Sum4/1, Switch5/1, Sterio camera + encoder/2(alpha_phi_dot)
  [r] -> Mux14/1, Sum5/1, Switch6/1, Sterio camera + encoder/4(r)
  [r_dot] -> Mux10/1, Sum6/1, Switch7/1, Sterio camera + encoder/5(r_dot)
  Sterio camera + encoder/2(alpha_phi_dot_est) -> Mux11/2, Sum4/2, Switch5/3
  Sterio camera + encoder/3(r_est) -> Sum5/2, Mux14/2, Switch6/3
  Switch2/1 -> [alpha_phi_est]
  Switch5/1 -> [alpha_phi_dot_est]
  Switch6/1 -> [r_est]
  Switch7/1 -> [r_dot_est]
  Sum3/1 -> [e_est_alpha_phi], "alpha  "/1
  [alpha_phi] -> Sum3/1, Switch2/1, Sterio camera + encoder/1("alpha, phi")
  Sterio camera + encoder/1(alpha_phi_est) -> Sum3/2, Switch2/3
  Sum4/1 -> "alpha dot "/1
  Sum5/1 -> [e_est_r], "r   "/1
  Sterio camera + encoder/4(r_dot_est) -> Mux10/2, Sum6/2, Switch7/3
  Sum6/1 -> "r dot  "/1
  [X_u_est] -> quadrotor position from relative buoy-UAV position/1(X_u)
  [Xdot_u_est] -> quadrotor position from relative buoy-UAV position/2(Xdot_u)
  [r_est] -> quadrotor position from relative buoy-UAV position/4(r)
  [r_dot_est] -> quadrotor position from relative buoy-UAV position/5(r_dot)
  [alpha_phi_est] -> quadrotor position from relative buoy-UAV position/7("alpha, phi")
  [alpha_phi_dot_est] -> quadrotor position from relative buoy-UAV position/8("(alpha, phi)_dot")
  quadrotor position from relative buoy-UAV position/2(Xdot_b) -> Mux4/2, Sum7/2, Switch9/3
  quadrotor position from relative buoy-UAV position/1(Xb) -> Sum9/2, Mux7/2, Switch8/3
  [alpha_phi_ddot] -> Switch10/1, Mux8/1, Sterio camera + encoder/3(alpha_phi_ddot)
  Sterio camera + encoder/5(alpha_phi_ddot_est) -> Mux8/2, Switch10/3
  Switch10/1 -> [alpha_phi_ddot_est]
  [Xdot_b] -> Mux4/1, Sum7/1, Switch9/1
  [alpha_phi_ddot_est] -> quadrotor position from relative buoy-UAV position/9("(alpha, phi)_ddot")
  [Xddot_u_est] -> quadrotor position from relative buoy-UAV position/3(Xddot_u)
  quadrotor position from relative buoy-UAV position/3(Xddot_b) -> Mux6/2, Sum8/2, Switch11/3
  [r_ddot] -> Mux9/1, Switch12/1, Sterio camera + encoder/6(r_ddot)
  Switch12/1 -> [r_ddot_est]
  Switch9/1 -> [Xdot_b_est]
  Switch11/1 -> [Xddot_b_est]
  Sum7/1 -> Xb_dot error/1
  Manual Switch/1 -> Switch10/2, Switch12/2, Switch8/2, Switch11/2, Switch9/2, Switch7/2, Switch6/2, Switch5/2, Switch2/2, Switch/2, Switch13/2, Switch4/2, Switch3/2, Switch1/2
  Sum8/1 -> "Xb_ddot error  "/1
  Sum9/1 -> [e_est_V], Xb error/1
  Switch8/1 -> [X_b_est]
  [X_b] -> Mux7/1, Sum9/1, Switch8/1
  Mux4/1 -> "Xb_ dot "/1
  Mux6/1 -> "Xb_ddot "/1
  [Xddot_b] -> Mux6/1, Sum8/1, Switch11/1
  [r_ddot_est] -> quadrotor position from relative buoy-UAV position/6(r_ddot)
  [X_ddot_u] -> Mux12/1, Sum10/1, Switch13/1, GPS/INS/3(X_ddot)
  Switch13/1 -> [Xddot_u_est]
  Mux7/1 -> "Xb "/1
  Mux8/1 -> "alpha ddot "/1
  Mux9/1 -> "r ddot   "/1
  Sterio camera + encoder/6(r_ddot_est) -> Mux9/2, Switch12/3
  Sum10/1 -> x ddot/1
  Mux10/1 -> r dot   1/1
  Mux11/1 -> alpha dot 2 2/1
  GPS/INS/5(X_ddot_est) -> Mux12/2, Sum10/2, Switch13/3
  Mux12/1 -> x ddot1/1
  Mux13/1 -> is coupled 1/1
  Mux14/1 -> r   1/1
  [r_est] -> Coupling detection by r/1(In1)
  [coupled_est] -> Coupling detection by r/2(In2)
  [T_est] -> Tension threshold/1
  Tension threshold/1 -> Data Type Conversion/1
  Data Type Conversion/1 -> Mux13/3
  Coupling detection by r/1(is coupled) -> Mux13/2
  [coupled] -> [coupled_est], Mux13/1

== system ML_UAV_3D_2/Subsystem ==
